simulink library "THB_fixed_mdot"  (R2018b)
settings: Solver=ode45  StartTime=0.0  StopTime=10.0  RelTol=1e-3  EnableMultiTasking=on
libraries: carnot x1
settings Model: Creator=lena.frank  LastModifiedBy=drhf
settings DataIOCC: LimitDataPoints=on  SaveFormat=Array  SignalLoggingSaveFormat=ModelDataLogs
settings OptimizationCC: ExpressionDepthLimit=2147483647  LifeSpan=inf
settings DebuggingCC: UnderspecifiedInitializationDetection=Classic  MergeDetectMultiDrivingBlocksExec=none  SolverPrmCheckMsg=warning  FcnCallInpInsideContextMsg=warning  StateNameClashWarn=warning  SFUnexpectedBacktrackingDiag=warning  SFNoUnconditionalDefaultTransitionDiag=warning  SFExecutionAtInitializationDiag=none
settings HardwareCC: ProdBitPerPointer=32  ProdBitPerSizeT=32  ProdBitPerPtrDiffT=32  ProdLargestAtomicFloat=None  ProdIntDivRoundTo=Undefined  ProdEndianess=Unspecified  ProdWordSize=32  ProdHWDeviceType=32-bit Generic
settings ModelReferenceCC: PropagateSignalLabelsOutOfModel=off
settings SFSimCC: SimUseLocalCustomCode=off
settings RTWCC: RTWUseLocalCustomCode=off
settings CodeAppCC: StateflowObjectComments=on
settings GRTTargetCC: TargetLangStandard=C89/C90 (ANSI)  GeneratePreprocessorConditionals=Disable all  CombineOutputUpdateFcns=off  GRTInterface=on
settings ConfigComp: CovMetricSettings=dw  CovHtmlReporting=on  CovSaveCumulativeToWorkspaceVar=on  CovSaveSingleToWorkspaceVar=on  CovExternalEMLEnable=off

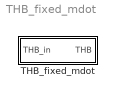
== system THB_fixed_mdot ==
  THB_fixed_mdot : Subsystem  InitFcn=load('THB.mat');  mask(set masssflow in THB){m=10/60}
      mask prompts: m "massflow in kg/s"
      mask help: Set a constant massflow in the thermo-hydraulic vector.
      mask Help: web(fullfile(path_carnot('help'),'THB_fixed_mdot.html'),'-helpbrowser')

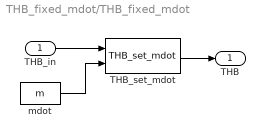
== system THB_fixed_mdot/THB_fixed_mdot ==
  THB_in : Inport
  THB_set_mdot : carnot/Source/Simple/THB_set_mdot
      settings: SourceProductName=Carnot
  mdot : Constant  Value=m
  THB : Outport
  wires:
  THB_set_mdot/1 -> THB/1
  THB_in/1 -> THB_set_mdot/1
  mdot/1 -> THB_set_mdot/2
